simulink model "Traffic_Lights"  (R2017b)
settings: Solver=VariableStepAuto  StartTime=0.0  StopTime=inf  RelTol=1e-3
settings Model: Creator=engdo  LastModifiedBy=engdo

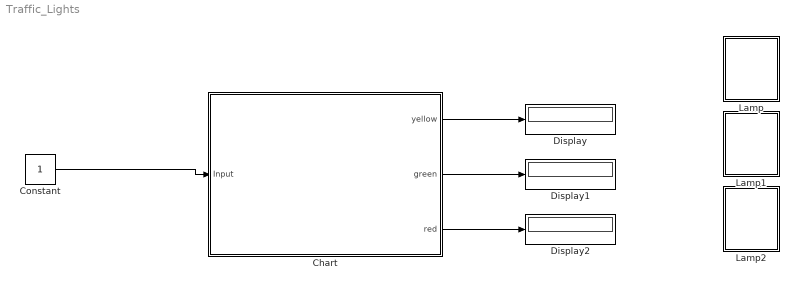
== system Traffic_Lights ==
  Chart : Stateflow chart  TreatAsAtomicUnit=on
  Constant : Constant
  Display : Display
  Display1 : Display
  Display2 : Display
  Lamp : Subsystem  DialogController=hmiCreateDDGDialog  IsWebBlock=on  mask(MWDashboardBlock){webBlockId=4e8607ef-3679-45e1-bbf2-9ef297ce5265, webBlockType=lamp, ShowInLibBrowser=on, ShowInitialText=on, HMISrcModelName=Traffic_Lights}
      mask prompts: webBlockType "WebBlock Type"; HMISrcModelName "Source Model"
      mask help: SimulinkHMI:dialogs:LampDialogDesc
      mask Help: helpview([docroot '/mapfiles/simulink.map'], 'hmi_lamp')
      mask Display:
      | if strcmp(get_param(bdroot(gcb),'BlockDiagramType'), 'library')
      |     image([(matlabroot) '/toolbox/simulink/hmi/icons/Lamp.png']);
      | end
  Lamp1 : Subsystem  DialogController=hmiCreateDDGDialog  IsWebBlock=on  mask(MWDashboardBlock){webBlockId=d5c0f31a-3ec1-4194-aaab-315fb586a4eb, webBlockType=lamp, ShowInLibBrowser=on, ShowInitialText=on, HMISrcModelName=Traffic_Lights}
      mask prompts: webBlockType "WebBlock Type"; HMISrcModelName "Source Model"
      mask help: SimulinkHMI:dialogs:LampDialogDesc
      mask Help: helpview([docroot '/mapfiles/simulink.map'], 'hmi_lamp')
      mask Display:
      | if strcmp(get_param(bdroot(gcb),'BlockDiagramType'), 'library')
      |     image([(matlabroot) '/toolbox/simulink/hmi/icons/Lamp.png']);
      | end
  Lamp2 : Subsystem  DialogController=hmiCreateDDGDialog  IsWebBlock=on  mask(MWDashboardBlock){webBlockId=f1518a10-f952-4b96-92d3-a942bbcdddf3, webBlockType=lamp, ShowInLibBrowser=on, ShowInitialText=on, HMISrcModelName=Traffic_Lights}
      mask prompts: webBlockType "WebBlock Type"; HMISrcModelName "Source Model"
      mask help: SimulinkHMI:dialogs:LampDialogDesc
      mask Help: helpview([docroot '/mapfiles/simulink.map'], 'hmi_lamp')
      mask Display:
      | if strcmp(get_param(bdroot(gcb),'BlockDiagramType'), 'library')
      |     image([(matlabroot) '/toolbox/simulink/hmi/icons/Lamp.png']);
      | end
  wires:
  Constant/1 -> Chart/1(Input)
  Chart/1(yellow) -> Display/1
  Chart/2(green) -> Display1/1
  Chart/3(red) -> Display2/1

== system Traffic_Lights/Lamp ==

== system Traffic_Lights/Lamp1 ==

== system Traffic_Lights/Lamp2 ==

== stateflow chart Traffic_Lights/Chart ==
  state TrafficLights
  state ON
  state OFF
  state entry__
    entry: red = 1;
    yellow = 0;
    green = 0;
    exit :
    red = 0;
    yellow = 0;
    green = 0
  state entry__1
    entry: red = 0;
    yellow = 1;
    green = 0;
    exit :
    red = 0;
    yellow = 0;
    green = 0
  state entry__2
    entry: red = 0;
    yellow = 0;
    green = 1;
    exit :
    red = 0;
    yellow = 0;
    green = 0
  (default) -> TrafficLights
  TrafficLights -> ON [order 1] : [Input == 1]
  TrafficLights -> OFF [order 2] : [Input == 0]
  ON -> entry__ : [Input == 1]
  entry__2 -> entry__ : after(120,sec)
  entry__ -> entry__1 : after(120,sec)
  entry__1 -> entry__2 : after(120,sec)
  data: Input input; yellow output; green output; red output
